simulink model "exp4"  (R2021b)
settings: Solver=VariableStepAuto  StartTime=0.0  StopTime=100  RelTol=1e-3
settings Model: Creator=ashir  LastModifiedBy=ashir

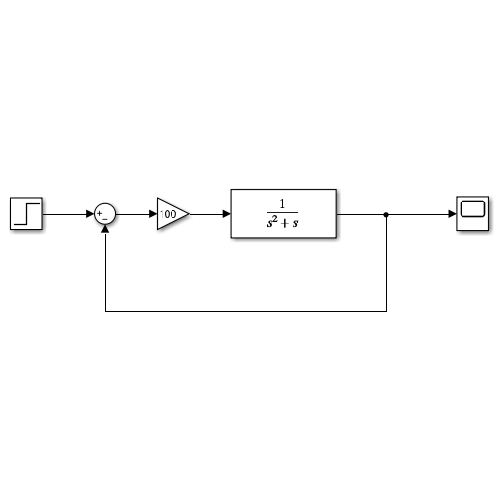
[thumbnail: Simulink's stored preview of the top-level diagram]
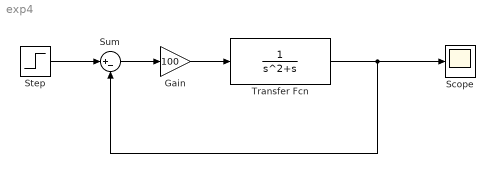
== system exp4 ==
  Gain : Gain  Gain=100
  Scope : Scope
  Step : Step  Time=0  SampleTime=0
  Sum : Sum  Inputs=|+-
  Transfer Fcn : TransferFcn  Denominator=[1 1 0]
  wires:
  Gain/1 -> Transfer Fcn/1
  Transfer Fcn/1 -> Sum/2, Scope/1
  Sum/1 -> Gain/1
  Step/1 -> Sum/1
